simulink model "TestBateria"  (R2023b)
settings: Solver=VariableStepAuto  StartTime=0.0  StopTime=10.0  RelTol=1e-3
libraries: arduinolib x1
settings Model: Creator=chaya  LastModifiedBy=chaya

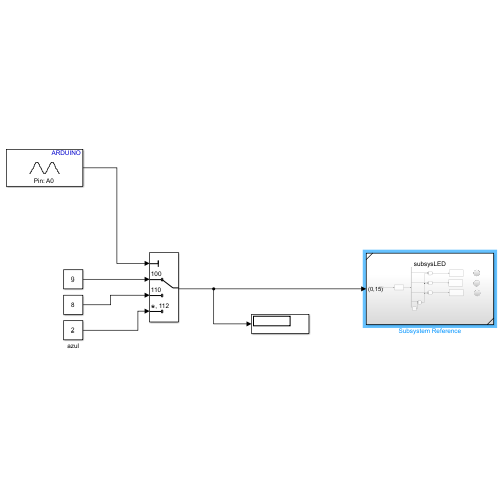
[thumbnail: Simulink's stored preview of the top-level diagram]
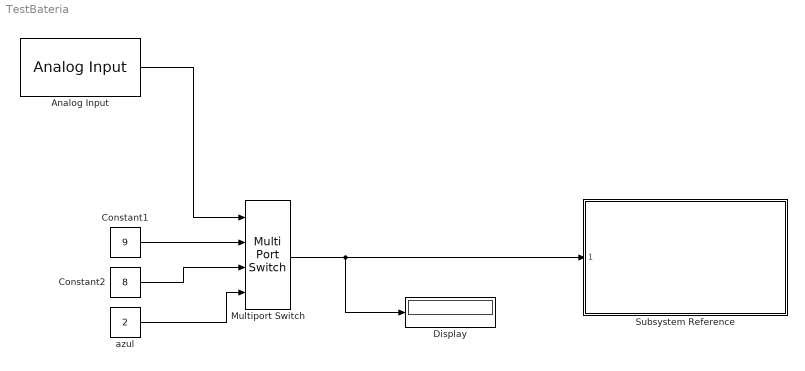
== system TestBateria ==
  Analog Input : arduinolib/Analog Input  pinNumber=0  ReadResultsOnly=off  ConversionTriggerSource=Software  ExternalTriggerType=uint32( 0 )  OutputDataType=uint16  EnableConversionCompleteNotify=off  EnableOuputStatus=off  SampleTime=0.01  blockPlatform=arduino
  Constant1 : Constant  Value=9
  Constant2 : Constant  Value=8
  Display : Display
  Multiport Switch : MultiPortSwitch  DataPortOrder=Specify indices  DataPortIndices={100,110,112}  SaturateOnIntegerOverflow=off  InputSameDT=off
  Subsystem Reference : Subsystem  ReferencedSubsystem=subsysLED
  azul : Constant  Value=2
  wires:
  Multiport Switch/1 -> Subsystem Reference/1, Display/1
  Analog Input/1 -> Multiport Switch/1
  Constant1/1 -> Multiport Switch/2
  Constant2/1 -> Multiport Switch/3
  azul/1 -> Multiport Switch/4
